simulink model "ASG_algorithm"  (R2024a)
settings: Solver=ode1  StartTime=0.0  StopTime=60  FixedStep=0.01  RelTol=1e-3
libraries: simulink x3
(part 3 of 3)

== matlab function ASG_algorithm/Subsystem1/AverageBlock7/MATLAB Function ==
  data: t input; t_plus_theta output; theta input
function t_plus_theta = fcn(t, theta)
t_plus_theta = 1/(t+theta);

== matlab function ASG_algorithm/MATLAB Function ==
  data: q_dot input; Q input; D_inv input; C_q input; g_q input; out output; drag_matrix input
function out = fcn(q_dot, Q, D_inv,C_q,g_q, drag_matrix)
out = zeros(6,1);
out=D_inv*((-C_q-drag_matrix)*q_dot-g_q+Q);

== matlab function ASG_algorithm/Subsystem1/AverageBlock8/MATLAB Function ==
  data: t input; t_plus_theta output; theta input
function t_plus_theta = fcn(t, theta)
t_plus_theta = 1/(t+theta);

== matlab function ASG_algorithm/Subsystem1/Enabled Subsystem1/MATLAB Function ==
  data: Qactual_0 output; Q_actual input; Q_desired input; Qdesired_0 output; Qdot_actual input; Qdotactual_0 output; Qdotdesired_0 output; Qdot_desired input
function [Qactual_0, Qdesired_0, Qdotactual_0, Qdotdesired_0]= fcn(Q_actual, Q_desired,  Qdot_actual, Qdot_desired)
Qactual_0 = Q_actual;
Qdesired_0 = Q_desired ;

Qdotactual_0 = Qdot_actual;
Qdotdesired_0 = Qdot_desired ;

== matlab function ASG_algorithm/Subsystem1/MATLAB Function15 ==
  data: delta3 input; s3 output; delta3_dot input; eta3 input; t input; theta3 input; a3x_average input; a3y_average input; a3z_average input; Z3 output; norm_s3 output; a3phi_average input; a3theta_average input; a3psi_average input; alpha input
function [s3, Z3, norm_s3]= fcn(delta3, delta3_dot, eta3,t,theta3, a3x_average, a3y_average, a3z_average , a3phi_average, a3theta_average, a3psi_average, alpha)
s3 = zeros(6,1);
Z3 = zeros(6,1);
norm_s3 =zeros(1,1);

Z3 = [a3x_average; a3y_average; a3z_average ;a3phi_average; a3theta_average; a3psi_average]; %[0; 0; 0; 0; 0; 0];
s3 = delta3_dot + (delta3+eta3)/(t+theta3) - Z3;    %+ [0; 0; 0; 0; 0; 0]
norm_s3 = norm(s3);

== matlab function ASG_algorithm/Subsystem1/AverageBlock10/MATLAB Function ==
  data: t input; t_plus_theta output; theta input
function t_plus_theta = fcn(t, theta)
t_plus_theta = 1/(t+theta);

== matlab function ASG_algorithm/Subsystem1/AverageBlock11/MATLAB Function ==
  data: t input; t_plus_theta output; theta input
function t_plus_theta = fcn(t, theta)
t_plus_theta = 1/(t+theta);

== matlab function ASG_algorithm/Subsystem1/AverageBlock9/MATLAB Function ==
  data: t input; t_plus_theta output; theta input
function t_plus_theta = fcn(t, theta)
t_plus_theta = 1/(t+theta);

== matlab function ASG_algorithm/Subsystem1/MATLAB Function22 ==
  data: z_vector input; delta32 output; D_inv input; C input; drag_matrix input; q_dot_signal input; G_q input; Kv input; R6 input; h0_omega input; omega_vector input; epsilon input; a3 output; alpha input; k32 input
function [delta32, a3] = fcn(z_vector, D_inv, C, drag_matrix, q_dot_signal, G_q, Kv, R6, h0_omega, omega_vector,epsilon, alpha, k32)
delta32 = zeros(1,1);
a3 = zeros(1,1);

delta32= -z_vector'*D_inv*(C+drag_matrix)*q_dot_signal - z_vector'*D_inv*G_q+ Kv*z_vector'*D_inv*R6*h0_omega*omega_vector;


F_d32 =1/2*norm(delta32)^2;

if F_d32 < epsilon
    a3 = zeros(1,1);
else
    a3 = (1-alpha)*k32*delta32;  %quite el signo /F_d3
end

== matlab function ASG_algorithm/Subsystem1/MATLAB Function23 ==
  data: Kv input; G322 output; R6 input; h0_omega input
function G322 = fcn(Kv, R6,h0_omega)
G322 = zeros(6,4);
G322 = 2*Kv*R6*h0_omega;

== matlab function ASG_algorithm/Subsystem1/MATLAB Function24 ==
  data: x input; h_x output; K11 input; K22 input; K33 input; larm input
function h_x = fcn(x, K11, K22, K33, larm)
h_x = zeros(6,4);

h_x =[0 0 0 0;
      0 0 0 0;
      x(1) x(2) x(3) x(4);
      larm*(K11'*x)';
      larm*(K22'*x)';
      larm*(K33'*x)'
      ];

== matlab function ASG_algorithm/Subsystem1/MATLAB Function25 ==
  data: x input; h_x output; K11 input; K22 input; K33 input; larm input
function h_x = fcn(x, K11, K22, K33, larm)
h_x = zeros(6,4);

h_x =[0 0 0 0;
      0 0 0 0;
      x(1) x(2) x(3) x(4);
      larm*(K11'*x)';
      larm*(K22'*x)';
      larm*(K33'*x)'
      ];

== matlab function ASG_algorithm/Subsystem1/MATLAB Function26 ==
  data: Jm input; Jm_inv output
function Jm_inv = fcn(Jm)
Jm_inv = 1/Jm;

== matlab function ASG_algorithm/Subsystem1/eta3 ==
  data: theta3 input; eta3 output; sum_result output; Qactual_0 input; Qdesired_0 input; Qdotactual_0 input; Qdotdesired_0 input
function [eta3, sum_result] = fcn(theta3, Qactual_0, Qdesired_0, Qdotactual_0, Qdotdesired_0)
eta3 = Qdesired_0 - Qactual_0 - theta3*(Qdotactual_0-Qdotdesired_0);

sum_result = theta3*(Qdotactual_0-Qdotdesired_0) + Qactual_0-Qdesired_0 + eta3;

== matlab function ASG_algorithm/Subsystem1/MATLAB Function27 ==
  data: x input; h_x output; K11 input; K22 input; K33 input; larm input
function h_x = fcn(x, K11, K22, K33, larm)
h_x = zeros(6,4);

h_x =[0 0 0 0;
      0 0 0 0;
      x(1) x(2) x(3) x(4);
      larm*(K11'*x)';
      larm*(K22'*x)';
      larm*(K33'*x)'
      ];

== matlab function ASG_algorithm/Subsystem1/MATLAB Function29 ==
  data: Kv input; z_vector input; G322 output; D_inv input; C input; R6 input; h0_omega input; drag_matrix input
function G322 = fcn(Kv, z_vector, D_inv, C, R6,h0_omega, drag_matrix)
G322 = zeros(1,4);
G322 = 2*Kv*z_vector'*D_inv*(-(C+drag_matrix)*D_inv*R6*h0_omega + R6*h0_omega);

== matlab function ASG_algorithm/MATLAB Function5 ==
  data: v_dot output; fv input; I_zero input; D_inv input; Q input; xi_subv input
function v_dot  = fcn(fv, I_zero, D_inv, Q, xi_subv)
v_dot = zeros(3,1);
v_dot=fv+I_zero*D_inv*Q+xi_subv;

== matlab function ASG_algorithm/Subsystem1/MATLAB Function30 ==
  data: Kv input; G311 output; R6 input; h0_omega input; R6_dot input; h0_omegadot input; t input; theta3 input; miu input
function G311 = fcn(Kv, R6,h0_omega, R6_dot, h0_omegadot, t, theta3, miu)
G311 = zeros(6,4);
G311 = 2*Kv*(R6*h0_omegadot +2*R6_dot*h0_omega + (1/(t+theta3) - 1/miu)*R6*h0_omega);

== matlab function ASG_algorithm/Subsystem1/MATLAB Function31 ==
  data: Kv input; R6_ddot input; h0_omega input; R6_dot input; t input; theta3 input; miu input; G311 output; R6 input
function G311 = fcn(Kv, R6_ddot,h0_omega, R6_dot, t, theta3, miu, R6)
G311 = zeros(6,4);
G311 = (Kv*R6_ddot + (1/(t+theta3) - 1/miu)*R6_dot + Kv*(1/(t+theta3) - 1/(t+theta3)^2)*R6)*h0_omega;

== matlab function ASG_algorithm/Subsystem1/MATLAB Function32 ==
  data: delta31 input; miu input; t input; theta3 input; Q_deseada input; zeta3 input; eta3 input; G313 output
function G313= fcn(delta31, miu, t, theta3, Q_deseada, zeta3, eta3)
G313 = zeros(6,1);
G313 = delta31*(1/(miu^2) - (1/(t+theta3)* 1/miu)) - Q_deseada/(t+theta3) -zeta3 + (Q_deseada -eta3)/(t+theta3)^2;

== matlab function ASG_algorithm/Subsystem1/MATLAB Function33 ==
  data: K11 output; K22 output; K33 output
function [K11, K22, K33 ]= fcn
K11= [0 0 0 0;
      0 -1 0 0;
      0  0 0 0;
      0 0 0 1];

K22= [1 0 0 0;
      0 0 0 0;
      0 0 -1 0;
      0 0 0 0] ;

K33= [1 0 0 0;
      0 -1 0 0;
      0  0 1 0;
      0 0 0 -1] ;

== matlab function ASG_algorithm/Subsystem1/MATLAB Function34 ==
  data: Kv input; z_vector input; G321 output; D_inv input; C input; R6 input; h0_omega input; drag_matrix input; h0_omegadot input; R6_dot input; theta3 input; t input
function G321 = fcn(Kv, z_vector, D_inv, C, R6,h0_omega, drag_matrix, h0_omegadot, R6_dot, theta3,t)
G321 = zeros(1,4);
G321 = 2*Kv*z_vector'*D_inv*(-(C+drag_matrix)*D_inv*(R6*h0_omegadot + 2*R6_dot*h0_omega)+2*R6_dot*h0_omega + R6*h0_omegadot+ (R6*h0_omega)/(t+theta3) );

== matlab function ASG_algorithm/Subsystem1/MATLAB Function35 ==
  data: Kv input; z_vector input; G320 output; D_inv input; C input; R6 input; h0_omega input; drag_matrix input; R6_dot input; theta3 input; t input; R6_ddot input; alpha input
function G320 = fcn(Kv, z_vector, D_inv, C, R6,h0_omega, drag_matrix, R6_dot, theta3,t, R6_ddot, alpha)
G320 = zeros(1,4);
G320 = Kv*z_vector'*(D_inv*(C+drag_matrix))^2*(D_inv*R6*h0_omega) + Kv*z_vector'*D_inv*(-(C+drag_matrix)*D_inv*R6_ddot*h0_omega + R6_ddot*h0_omega - (R6*h0_omega)/(t+theta3)^2 + (-(C+drag_matrix)*D_inv*R6*h0_omega + R6_dot*h0_omega + (1-alpha)*R6*h0_omega)/(t+theta3));

== matlab function ASG_algorithm/Subsystem/MATLAB Function2 ==
  data: Q_star input; Q_dot_star output; miu input; miu2 input; u1 input
function Q_dot_star = fcn(Q_star, miu,miu2, u1)
miu_matrix = [miu*eye(3,3) zeros(3,3); zeros(3,3) miu2*eye(3,3)];
Q_dot_star =pinv(miu_matrix)*(u1-Q_star);
%Q_dot_star = [Q_dot_star1(1:2); abs(Q_dot_star1(3)); Q_dot_star1(4:6) ];

== matlab function ASG_algorithm/Subsystem1/MATLAB Function36 ==
  data: z_vector input; D_inv input; C input; drag_matrix input; theta3 input; t input; alpha input; q_dot input; G_q input; eta3 input; G323 output
function G323 = fcn( z_vector, D_inv, C, drag_matrix, theta3,t, alpha, q_dot, G_q,eta3)
G323 = zeros(1,1);
G323 = z_vector'*(D_inv*(C+drag_matrix))^2*(-D_inv*(C+drag_matrix)*q_dot - D_inv*G_q) + z_vector'*D_inv*( ((C+drag_matrix)*q_dot + G_q)/(t+theta3)^2 + ((C+drag_matrix)*(D_inv*(C+drag_matrix)*q_dot + D_inv*G_q))/(t+theta3) + ((1-alpha)*( -C*q_dot -drag_matrix*q_dot - G_q))/(t+theta3) - eta3/(t+theta3)^2);

== matlab function ASG_algorithm/Subsystem1/MATLAB Function37 ==
  data: delta32 input; s32 output; delta32_dot input; eta32 input; t input; theta3 input; a3x_average input; Z32 output; norm_s3 output; alpha input
function [s32, Z32, norm_s3]= fcn(delta32, delta32_dot, eta32,t,theta3, a3x_average, alpha)
s32 = zeros(1,1);
Z32 = zeros(1,1);
norm_s3 = zeros(1,1);

Z32 = a3x_average; %[0; 0; 0; 0; 0; 0];
s32 = delta32_dot + (delta32+eta32)/(t+theta3) - Z32;    %+ [0; 0; 0; 0; 0; 0]
norm_s3 = norm(s32);

== matlab function ASG_algorithm/Subsystem1/eta4 ==
  data: theta3 input; delta32_0 input; eta3 output; sum_result output; delta32_dot0 input
function [eta3, sum_result] = fcn(theta3, delta32_0, delta32_dot0)
eta3 = zeros(1,1);

eta3 = -theta3*delta32_dot0 - delta32_0;
sum_result = theta3*delta32_dot0 + delta32_0 + eta3;

== matlab function ASG_algorithm/Subsystem1/Enabled Subsystem2/MATLAB Function ==
  data: delta32_0 output; delta32 input; delta32_dot input; delta32_dot_0 output
function [delta32_0, delta32_dot_0]= fcn(delta32, delta32_dot)
delta32_0 = delta32;
delta32_dot_0 = delta32_dot ;

== matlab function ASG_algorithm/Subsystem1/MATLAB Function39 ==
  data: u input; derivada output; u_delay input
function derivada = fcn(u, u_delay)
delta_t= 0.001;
derivada = (u - u_delay)/delta_t;

== matlab function ASG_algorithm/Subsystem1/MATLAB Function40 ==
  data: u input; derivada output; u_delay input
function derivada = fcn(u, u_delay)
delta_t= 0.001;
derivada = (u - u_delay)/delta_t;

== matlab function ASG_algorithm/Subsystem1/MATLAB Function38 ==
  data: S31 input; S3 output; S32 input
function S3 = fcn(S31, S32)
S3 = zeros(7,1);
S3 = [S31;S32];

== matlab function ASG_algorithm/Subsystem1/AverageBlock12/MATLAB Function ==
  data: t input; t_plus_theta output; theta input
function t_plus_theta = fcn(t, theta)
t_plus_theta = 1/(t+theta);

== matlab function ASG_algorithm/Subsystem1/AverageBlock13/MATLAB Function ==
  data: t input; t_plus_theta output; theta input
function t_plus_theta = fcn(t, theta)
t_plus_theta = 1/(t+theta);

== matlab function ASG_algorithm/Subsystem1/AverageBlock14/MATLAB Function ==
  data: t input; t_plus_theta output; theta input
function t_plus_theta = fcn(t, theta)
t_plus_theta = 1/(t+theta);

== matlab function ASG_algorithm/MATLAB Function10 ==
  data: I_zero input; fv output; D_inv input; C input; v input; omega input; g_q input; kf_c0 input; drag_matrix input
function fv = fcn(I_zero, D_inv, C, v, omega, g_q, kf_c0,drag_matrix)
fv=zeros(3,1);
fv = -I_zero*D_inv*(C+drag_matrix)*[v;omega]-I_zero*D_inv*(g_q);

== matlab function ASG_algorithm/Subsystem1/MATLAB Function41 ==
  data: G312 input; G322 input; gamma input; n3 input; omegaddot output
function omegaddot = fcn(G312, G322, gamma,n3)
omegaddot = zeros(4,1);
omegaddot = gamma*[G312;G322]'*n3;

== matlab function ASG_algorithm/Subsystem1/MATLAB Function42 ==
  data: n3 input; s3 input; k3 input; G312 input; s31 input; s32 input; G322 input; gamma output; h3 input
function gamma = fcn(n3, s3, k3, G312, s31, s32, G322, h3)
gamma =zeros(1,1);
gamma = -(n3'*(h3+ k3*sign(s3)))/(norm([G312;G322]'*n3)^2+0.001 );

== matlab function ASG_algorithm/Subsystem1/MATLAB Function43 ==
  data: G311 input; h31 output; G310 input; G313 input; omega_dot input; omega input; G321 input; G320 input; G323 input; h32 output; h3 output
function [h31, h32, h3] = fcn(G311, G310, G313, omega_dot, omega, G321, G320, G323)
h31 = zeros(6,1);
h32 = zeros(1,1);
h3 = zeros(7,1);

h31 = G311*omega_dot + G310*omega + G313;
h32 = G321*omega_dot + G320*omega + G323;

h3=[h31;h32];

== matlab function ASG_algorithm/Subsystem1/MATLAB Function44 ==
  data: h0_omega input; y output; omega input; kv input
function y = fcn(h0_omega,omega,kv)
y = zeros(6,1);
y = kv*h0_omega*omega;

== matlab function ASG_algorithm/MATLAB Function45 ==
  data: v_lin input; q_dot_signal output; v_ang input
function q_dot_signal  = fcn(v_lin, v_ang)
q_dot_signal = zeros(6,1);

q_dot_signal =[v_lin;v_ang];

== matlab function ASG_algorithm/Subsystem1/MATLAB Function46 ==
  data: Fb input; Q_costructed output; R6 input
function Q_costructed = fcn(Fb, R6)
Q_costructed = R6*Fb;

== matlab function ASG_algorithm/Subsystem1/MATLAB Function47 ==
  data: s3 input; n3 output
function n3 = fcn(s3)
n3 = s3/(norm(s3)+0.01);

== matlab function ASG_algorithm/MATLAB Function1 ==
  data: Kv input; mixer output; Km input; mixer_inv output
function [mixer, mixer_inv] = fcn(Kv, Km)
mixer= zeros(4,4);
mixer_inv= zeros(4,4); 

mixer = [Kv Kv Kv Kv ;
         0 -Kv 0 Kv;
         Kv 0 -Kv 0;
         Km -Km Km -Km
    ];
mixer_inv= pinv(mixer);

== matlab function ASG_algorithm/MATLAB Function26 ==
  data: Jm input; Jm_inv output
function Jm_inv = fcn(Jm)
Jm_inv = 1/Jm;

== matlab function ASG_algorithm/MATLAB Function2 ==
  data: mixer_inv input; rotors_vel output; control4x1 input
function rotors_vel = fcn(mixer_inv, control4x1)
rotors_vel= zeros(4,1);
rotors_vel = mixer_inv*control4x1;

== matlab function ASG_algorithm/MATLAB Function13 ==
  data: Q input; Q_6X1 output; R_inv input
function Q_6X1 = fcn(Q, R_inv)
Q_6X1 = zeros(6,1);

aux1 = R_inv*Q(1:3);
Q_6X1 = [aux1;Q(4:6)];

== matlab function ASG_algorithm/MATLAB Function15 ==
  data: angles_vector input; R output; anglesdot_vector input; R_dot output; R_ddot output; anglesddot_vector input; R_inv output
function [R, R_dot, R_ddot, R_inv]= fcn(angles_vector, anglesdot_vector, anglesddot_vector)
R = zeros(3,3);
R_dot = zeros(3,3);
R_ddot= zeros(3,3);
R_inv= zeros(3,3);



phi = angles_vector(1);
theta = angles_vector(2);
psi = angles_vector(3);


phi_dot = anglesdot_vector(1);
theta_dot = anglesdot_vector(2);
psi_dot = anglesdot_vector(3);

phi_ddot = anglesddot_vector(1);
theta_ddot = anglesddot_vector(2);
psi_ddot = anglesddot_vector(3);


 R = [ cos(theta)*cos(psi), cos(psi)*sin(phi)*sin(theta) - cos(phi)*sin(psi) , sin(phi)*sin(psi)+cos(phi)*cos(psi)*sin(theta);
       cos(theta)*sin(psi), cos(phi)*cos(psi) + sin(phi)*sin(theta)*sin(psi) , cos(phi)*sin(theta)*sin(psi)-cos(psi)*sin(phi);
       -sin(theta) , cos(theta)*sin(phi) , cos(phi)*cos(theta)];

R_inv=pinv(R);

 R_dot = -[0      -psi_dot theta_dot;
           psi_dot 0    -phi_dot;
           -theta_dot phi_dot 0 ] * R;

 matrix_aux =  [0      -psi_dot theta_dot;
           psi_dot 0    -phi_dot;
           -theta_dot phi_dot 0 ];

 R_ddot = (-[0      -psi_ddot theta_ddot;
           psi_ddot 0    -phi_ddot;
           -theta_ddot phi_ddot 0 ]   +  matrix_aux^2 )* R;

== matlab function ASG_algorithm/MATLAB Function22 ==
  data: Q6x1 input; Q4x1 output
function Q4x1 = fcn(Q6x1)
Q4x1 = zeros(4,1);
Q4x1 = Q6x1(3:6);

== matlab function ASG_algorithm/MATLAB Function23 ==
  data: R input; Q_actual output; mixer input; rotors_vel4x1 input
function Q_actual = fcn(R, mixer, rotors_vel4x1)
Q_actual= zeros(6,1);
aux=mixer*rotors_vel4x1;
Fb = R*[0;0;aux(1)];
Q_actual=[Fb;aux(2:4)];

== matlab function ASG_algorithm/MATLAB Function24 ==
  data: M input; Fz output; g input; Ka input; q_dot input; q_ddot input; theta_actual input; Q6 input; Q4 output
function [Fz, Q4 ]= fcn(M, g, Ka, q_dot, q_ddot, theta_actual,Q6)
% m z_ddot + mg - Fa = R Fz_body
% RFb = Fz

Q4 = zeros(4,1);
Fz = zeros(1,1);

Fz = (M*(q_ddot(3)+g)+ Ka*q_dot(3))/(cos(theta_actual(1))*cos(theta_actual(2)));
%Fz = (M*(q_ddot(3)+g))/(cos(theta_actual(1))*cos(theta_actual(2)));
Q4 = [Fz;Q6(4:6)];

== matlab function ASG_algorithm/MATLAB Function11 ==
  data: zero_I input; fw output; D_inv input; C input; v input; omega input; g_q input; drag_matrix input; Kf_c0 input
function fw = fcn(zero_I, D_inv, C, v, omega, g_q, drag_matrix, Kf_c0)
fw=zeros(3,1);
fw =-zero_I*D_inv*(C+drag_matrix)*[v;omega]-zero_I*D_inv*(g_q);

== matlab function ASG_algorithm/MATLAB Function25 ==
  data: v_lin input; q_dot_signal output; v_ang input
function q_dot_signal  = fcn(v_lin, v_ang)
q_dot_signal = zeros(6,1);

q_dot_signal =[v_lin;v_ang];

== matlab function ASG_algorithm/MATLAB Function27 ==
  data: Kv input; Km output; porcent_force input
function Km = fcn(Kv, porcent_force)
%porcent_force [0.01 - 0.05]
Km = Kv*porcent_force;
